simulink model "lfo_multiplier"  (R2018a)
settings: Solver=FixedStepDiscrete  StartTime=0.0  StopTime=30.0  RelTol=1e-3
settings Model: Creator=Lu  LastModifiedBy=Lu
settings DataIOCC: SaveOutput=off  SaveTime=off
settings OptimizationCC: BlockReduction=off  ConditionallyExecuteInputs=off  DefaultParameterBehavior=Inlined
settings DebuggingCC: AlgebraicLoopMsg=error  SingleTaskRateTransMsg=error
settings HardwareCC: ProdBitPerPointer=32  ProdBitPerSizeT=32  ProdBitPerPtrDiffT=32  ProdLargestAtomicFloat=None  ProdIntDivRoundTo=Undefined  ProdEndianess=Unspecified  ProdWordSize=32  ProdHWDeviceType=ASIC/FPGA->ASIC/FPGA  TargetBitPerPointer=64  TargetBitPerSizeT=64  TargetBitPerPtrDiffT=64  TargetLongLongMode=on  TargetIntDivRoundTo=Zero  TargetEndianess=LittleEndian  TargetWordSize=64  TargetHWDeviceType=Custom Processor->MATLAB Host Computer  ProdEqTarget=off

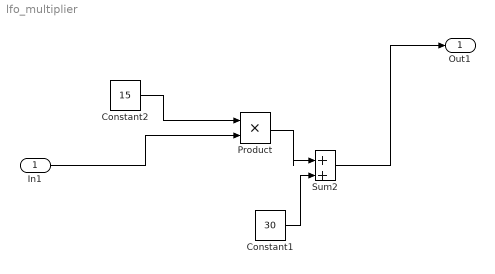
== system lfo_multiplier ==
  In1 : Inport  OutDataTypeStr=fixdt(1,16,14)  PortDimensions=[1 1]  SampleTime=[2.2675736961451248e-05,0]
  Constant1 : Constant  Value=30  OutDataTypeStr=fixdt(1,16)
  Constant2 : Constant  Value=15  OutDataTypeStr=fixdt(1,16)
  Product : Product  SaturateOnIntegerOverflow=on
  Sum2 : Sum  Inputs=|++  AccumDataTypeStr=fixdt(1,16,0)  RndMeth=Ceiling  SaturateOnIntegerOverflow=on
  Out1 : Outport  OutDataTypeStr=int16  PortDimensions=[1 1]  SampleTime=[2.2675736961451248e-05,0]
  wires:
  Constant1/1 -> Sum2/2
  Product/1 -> Sum2/1
  In1/1 -> Product/2
  Constant2/1 -> Product/1
  Sum2/1 -> Out1/1
